simulink library "VolumeMute"  (R2022b)
settings: Solver=VariableStepAuto  StartTime=0.0  StopTime=10.0  RelTol=1e-3
libraries: NonEntGainCalcBtc x4, NonEntVncAppliedBtc x4, FeaturePath x4, MuteBtc x4, AnnVolumeBtc x4, AnnouncementLevelDetection x1, HandyTextFile x1, RTC x1
settings Model: Creator=ak1044356  LastModifiedBy=sa1045272
settings SolverCC: AlgebraicLoopSolver=TrustRegion
settings DebuggingCC: UnconnectedInputMsg=warning  UnconnectedOutputMsg=warning  UnconnectedLineMsg=warning  SFMachineParentedDataDiag=warning  ArithmeticOperatorsInVariantConditions=warning
settings ModelReferenceCC: EnableRefExpFcnMdlSchedulingChecks=on
settings SFSimCC: CustomCodeUndefinedFunction=UseInterfaceOnly

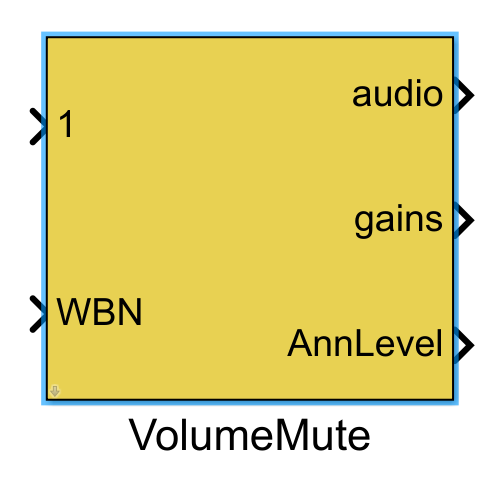
[thumbnail: Simulink's stored preview of the top-level diagram]
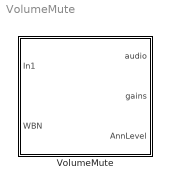
== system VolumeMute ==
  VolumeMute : Subsystem  mask{Config=[]}
      mask prompts: Config "VolumeMuteConfig"
      mask init:
      | blkh=gcbh;
      | Config=BTConfig.Assert(blkh,Config);
      | 
      | Config.Validate();
      | Config.DoMaskInit(blkh);

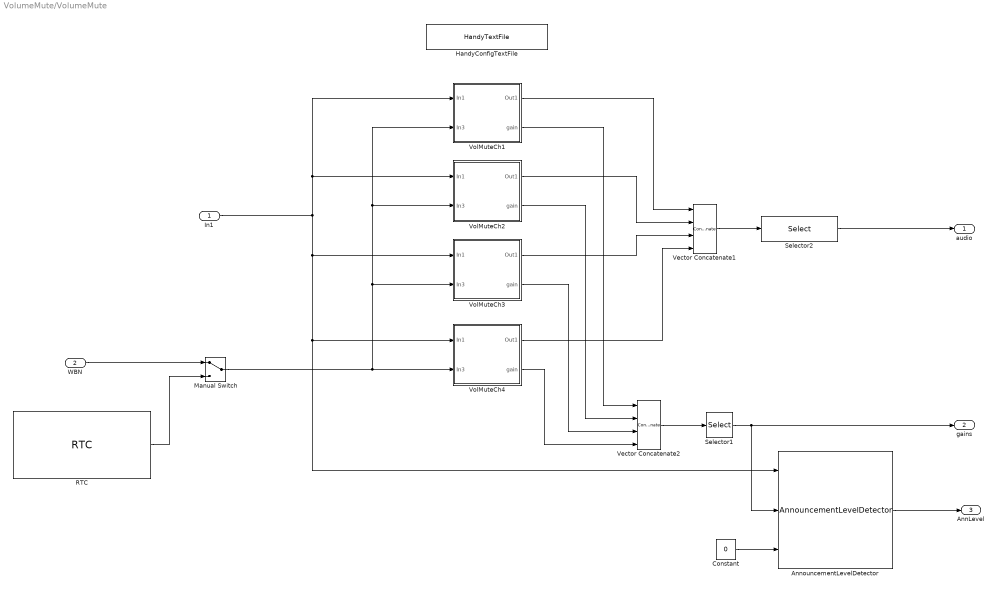
== system VolumeMute/VolumeMute ==
  In1 : Inport
  WBN : Inport  Port=2
  AnnouncementLevelDetector : AnnouncementLevelDetection/AnnouncementLevelDetector  vm=VolumeMuteConfig  DefaultFlag=off  Config=Config.AnnouncementLevelDetector
  Constant : Constant  Value=0
  HandyConfigTextFile : HandyTextFile/HandyTextFile  TemplateSource=Config  FileSuffix=File  OpenDialogOnLoad=off  UseThisBlockName=off  AddGrandParentNamePrefix=off  TheDefaultText=% $(FILENAME) $(PREFIX) $(SUFFIX)  ShowInLibBrowser=on
      settings: SourceProductName=Bose Talaria
  Manual Switch : ManualSwitch
  RTC : RTC/RTC  REQ_Priority=RTC_Mask.NormalPriority  RequestAtInit=off  EnableRequest=off  REQElemName1=NoiseSig  REQElemType1=single  REQElemWidth1=1  REQElemInitial1=NEAR_initial_noise_level  REQElemType2=uint32  REQElemWidth2=1  REQElemInitial2=[]  REQElemType3=uint32  REQElemWidth3=1  REQElemInitial3=[]  REQElemType4=uint32  REQElemWidth4=1  REQElemInitial4=[]  REQElemType5=uint32  REQElemWidth5=1  REQElemInitial5=[]  REQElemType6=uint32  REQElemWidth6=1  REQElemInitial6=[]  REQElemType7=uint32  REQElemWidth7=1  REQElemInitial7=[]  REQElemType8=uint32  REQElemWidth8=1  REQElemInitial8=[]  REQElemType9=uint32  REQElemWidth9=1  REQElemInitial9=[]  REQElemType10=uint32  REQElemWidth10=1  REQElemInitial10=[]  EnableResponse=off  EnableRSP_StatusIn=off  RSPElemType1=uint32  RSPElemWidth1=1  RSPElemType2=uint32  RSPElemWidth2=1  RSPElemType3=uint32  RSPElemWidth3=1  RSPElemType4=uint32  RSPElemWidth4=1  RSPElemType5=uint32  RSPElemWidth5=1  RSPElemType6=uint32  RSPElemWidth6=1  RSPElemType7=uint32  RSPElemWidth7=1  RSPElemType8=uint32  RSPElemWidth8=1  RSPElemType9=uint32  RSPElemWidth9=1  RSPElemType10=uint32  RSPElemWidth10=1  EnableNotification=off  EnableNTF_PrepTrig=off  NTFElemType1=uint32  NTFElemWidth1=1  NTFElemType2=uint32  NTFElemWidth2=1  NTFElemType3=uint32  NTFElemWidth3=1  NTFElemType4=uint32  NTFElemWidth4=1  NTFElemType5=uint32  NTFElemWidth5=1  NTFElemType6=uint32  NTFElemWidth6=1  NTFElemType7=uint32  NTFElemWidth7=1  NTFElemType8=uint32  NTFElemWidth8=1  NTFElemType9=uint32  NTFElemWidth9=1  NTFElemType10=uint32  NTFElemWidth10=1  MaskMessageName=AnnNoiseLevel
      settings: SourceProductName=Bose Talaria
  Selector1 : Selector  NumberOfDimensions=2  InputPortWidth=3  IndexOptions=Select all,Index vector (dialog)  Indices=[1 3],1:Config.AnnChannelCount  OutputSizes=1,1
  Selector2 : Selector  NumberOfDimensions=2  InputPortWidth=3  IndexOptions=Select all,Index vector (dialog)  Indices=[1 3],1:Config.AnnChannelCount  OutputSizes=1,1
  Vector Concatenate1 : Concatenate  NumInputs=4  Mode=Multidimensional array  ConcatenateDimension=2
  Vector Concatenate2 : Concatenate  NumInputs=4  Mode=Multidimensional array  ConcatenateDimension=2
  VolMuteCh1 : Subsystem
  VolMuteCh2 : Subsystem
  VolMuteCh3 : Subsystem
  VolMuteCh4 : Subsystem
  audio : Outport  VectorParamsAs1DForOutWhenUnconnected=off
  gains : Outport  Port=2
  AnnLevel : Outport  Port=3
  wires:
  WBN/1 -> Manual Switch/1
  RTC/1 -> Manual Switch/2
  AnnouncementLevelDetector/1 -> AnnLevel/1
  Constant/1 -> AnnouncementLevelDetector/3
  Selector1/1 -> AnnouncementLevelDetector/2, gains/1
  VolMuteCh4/2(gain) -> Vector Concatenate2/4
  VolMuteCh3/2(gain) -> Vector Concatenate2/3
  VolMuteCh2/2(gain) -> Vector Concatenate2/2
  VolMuteCh1/2(gain) -> Vector Concatenate2/1
  Vector Concatenate2/1 -> Selector1/1
  Manual Switch/1 -> VolMuteCh4/2(In3), VolMuteCh3/2(In3), VolMuteCh2/2(In3), VolMuteCh1/2(In3)
  Selector2/1 -> audio/1
  Vector Concatenate1/1 -> Selector2/1
  In1/1 -> VolMuteCh2/1(In1), VolMuteCh1/1(In1), VolMuteCh3/1(In1), AnnouncementLevelDetector/1, VolMuteCh4/1(In1)
  VolMuteCh1/1(Out1) -> Vector Concatenate1/1
  VolMuteCh3/1(Out1) -> Vector Concatenate1/3
  VolMuteCh4/1(Out1) -> Vector Concatenate1/4
  VolMuteCh2/1(Out1) -> Vector Concatenate1/2

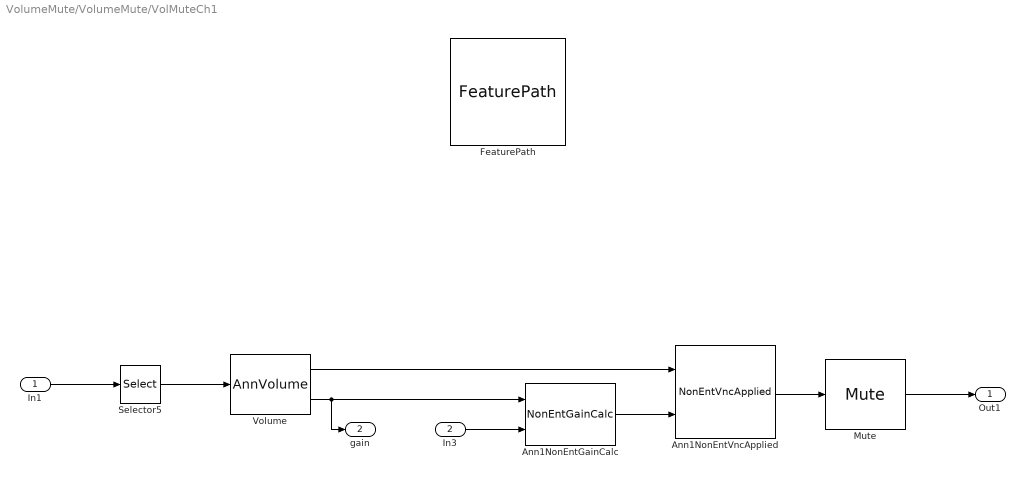
== system VolumeMute/VolumeMute/VolMuteCh1 ==
  In1 : Inport
  In3 : Inport  Port=2
  Ann1NonEntGainCalc : NonEntGainCalcBtc/NonEntGainCalc  Config=Config.Ann1NonEntGainCalc  FeatureName=Ann1NonEntGainCalc
      settings: SourceProductName=Bose Blocklib
  Ann1NonEntVncApplied : NonEntVncAppliedBtc/NonEntVncApplied  Config=Config.Ann1NonEntVncApplied  FeatureName=Ann1NonEntVncApplied
      settings: SourceProductName=Bose Blocklib
  FeaturePath : FeaturePath/FeaturePath  FeatureName=Ann1  IsGroup=off  GroupNumber=-1  IsModule=off  TriggerInit=[270 -291 385 -184]
      settings: SourceProductName=Bose Talaria
  Mute : MuteBtc/Mute  Config=Config.Ann1Mute  FeatureName=Ann1Mute
      settings: SourceProductName=Bose Blocklib
  Selector5 : Selector  NumberOfDimensions=2  InputPortWidth=3  IndexOptions=Select all,Index vector (dialog)  Indices=[1 3],1  OutputSizes=1,1
  Volume : AnnVolumeBtc/AnnVolume  FeatureName=Ann1Volume  Config=Config.Ann1Volume  TriggerInit=[50 25 130 85]
      settings: SourceProductName=Bose Blocklib
  Out1 : Outport  VectorParamsAs1DForOutWhenUnconnected=off
  gain : Outport  Port=2
  wires:
  Mute/1 -> Out1/1
  In1/1 -> Selector5/1
  Selector5/1 -> Volume/1
  In3/1 -> Ann1NonEntGainCalc/2
  Volume/1 -> Ann1NonEntVncApplied/1
  Volume/2 -> Ann1NonEntGainCalc/1, gain/1
  Ann1NonEntVncApplied/1 -> Mute/1
  Ann1NonEntGainCalc/1 -> Ann1NonEntVncApplied/2

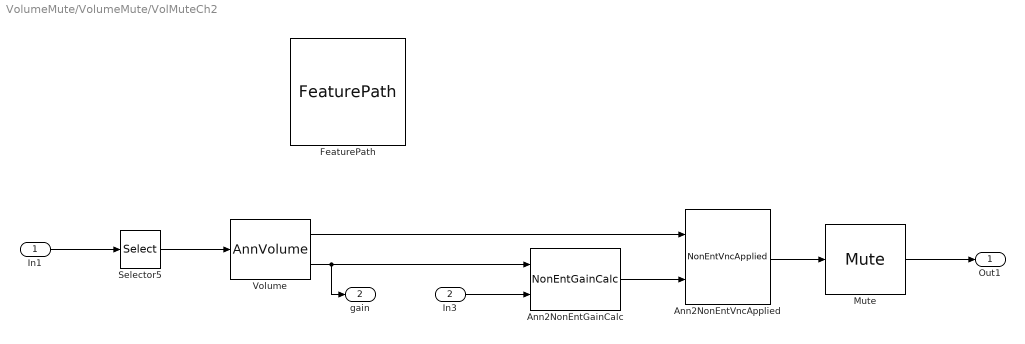
== system VolumeMute/VolumeMute/VolMuteCh2 ==
  In1 : Inport
  In3 : Inport  Port=2
  Ann2NonEntGainCalc : NonEntGainCalcBtc/NonEntGainCalc  Config=Config.Ann2NonEntGainCalc  FeatureName=Ann2NonEntGainCalc
      settings: SourceProductName=Bose Blocklib
  Ann2NonEntVncApplied : NonEntVncAppliedBtc/NonEntVncApplied  Config=Config.Ann2NonEntVncApplied  FeatureName=Ann2NonEntVncApplied
      settings: SourceProductName=Bose Blocklib
  FeaturePath : FeaturePath/FeaturePath  FeatureName=Ann2  IsGroup=off  GroupNumber=-1  IsModule=off  TriggerInit=[60 -206 175 -99]
      settings: SourceProductName=Bose Talaria
  Mute : MuteBtc/Mute  Config=Config.Ann2Mute  FeatureName=Ann2Mute
      settings: SourceProductName=Bose Blocklib
  Selector5 : Selector  NumberOfDimensions=2  InputPortWidth=3  IndexOptions=Select all,Index vector (dialog)  Indices=[1 3],min(2, Config.AnnChannelCount)  OutputSizes=1,1
  Volume : AnnVolumeBtc/AnnVolume  FeatureName=Ann2Volume  Config=Config.Ann2Volume  TriggerInit=[0 -25 80 35]
      settings: SourceProductName=Bose Blocklib
  Out1 : Outport  VectorParamsAs1DForOutWhenUnconnected=off
  gain : Outport  Port=2
  wires:
  Ann2NonEntGainCalc/1 -> Ann2NonEntVncApplied/2
  Ann2NonEntVncApplied/1 -> Mute/1
  Volume/2 -> Ann2NonEntGainCalc/1, gain/1
  Volume/1 -> Ann2NonEntVncApplied/1
  Selector5/1 -> Volume/1
  In1/1 -> Selector5/1
  In3/1 -> Ann2NonEntGainCalc/2
  Mute/1 -> Out1/1

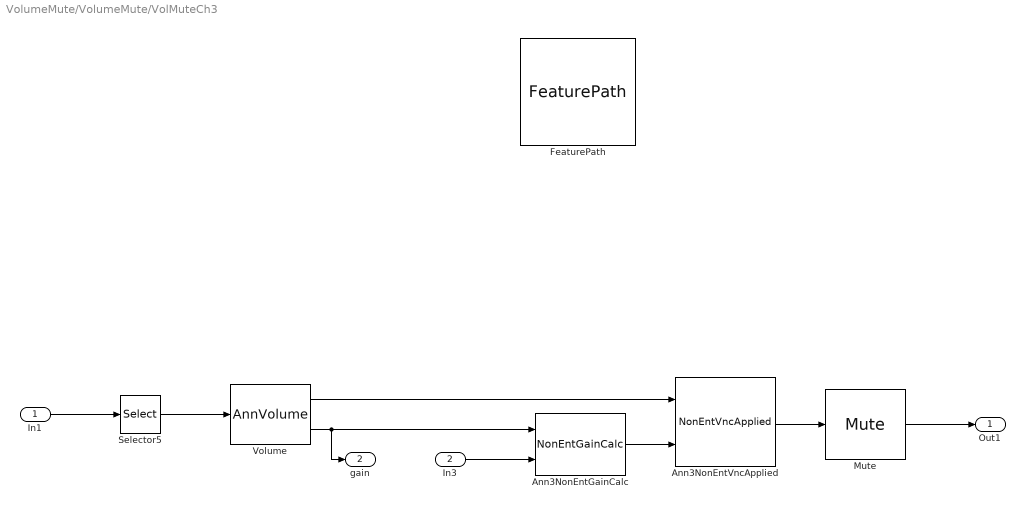
== system VolumeMute/VolumeMute/VolMuteCh3 ==
  In1 : Inport
  In3 : Inport  Port=2
  Ann3NonEntGainCalc : NonEntGainCalcBtc/NonEntGainCalc  Config=Config.Ann3NonEntGainCalc  FeatureName=Ann3NonEntGainCalc
      settings: SourceProductName=Bose Blocklib
  Ann3NonEntVncApplied : NonEntVncAppliedBtc/NonEntVncApplied  Config=Config.Ann3NonEntVncApplied  FeatureName=Ann3NonEntVncApplied
      settings: SourceProductName=Bose Blocklib
  FeaturePath : FeaturePath/FeaturePath  FeatureName=Ann3  IsGroup=off  GroupNumber=-1  IsModule=off  TriggerInit=[265 -336 380 -229]
      settings: SourceProductName=Bose Talaria
  Mute : MuteBtc/Mute  Config=Config.Ann3Mute  FeatureName=Ann3Mute
      settings: SourceProductName=Bose Blocklib
  Selector5 : Selector  NumberOfDimensions=2  InputPortWidth=3  IndexOptions=Select all,Index vector (dialog)  Indices=[1 3],min(3, Config.AnnChannelCount)  OutputSizes=1,1
  Volume : AnnVolumeBtc/AnnVolume  FeatureName=Ann3Volume  Config=Config.Ann3Volume  TriggerInit=[815 415 895 475]
      settings: SourceProductName=Bose Blocklib
  Out1 : Outport  VectorParamsAs1DForOutWhenUnconnected=off
  gain : Outport  Port=2
  wires:
  Ann3NonEntGainCalc/1 -> Ann3NonEntVncApplied/2
  Ann3NonEntVncApplied/1 -> Mute/1
  Volume/2 -> Ann3NonEntGainCalc/1, gain/1
  Volume/1 -> Ann3NonEntVncApplied/1
  Selector5/1 -> Volume/1
  In1/1 -> Selector5/1
  In3/1 -> Ann3NonEntGainCalc/2
  Mute/1 -> Out1/1

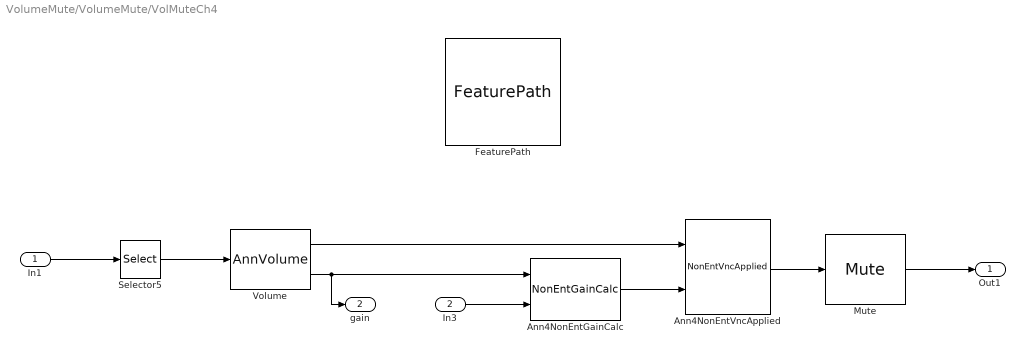
== system VolumeMute/VolumeMute/VolMuteCh4 ==
  In1 : Inport
  In3 : Inport  Port=2
  Ann4NonEntGainCalc : NonEntGainCalcBtc/NonEntGainCalc  Config=Config.Ann4NonEntGainCalc  FeatureName=Ann4NonEntGainCalc
      settings: SourceProductName=Bose Blocklib
  Ann4NonEntVncApplied : NonEntVncAppliedBtc/NonEntVncApplied  Config=Config.Ann4NonEntVncApplied  FeatureName=Ann4NonEntVncApplied
      settings: SourceProductName=Bose Blocklib
  FeaturePath : FeaturePath/FeaturePath  FeatureName=Ann4  IsGroup=off  GroupNumber=-1  IsModule=off  TriggerInit=[235 -186 350 -79]
      settings: SourceProductName=Bose Talaria
  Mute : MuteBtc/Mute  Config=Config.Ann4Mute  FeatureName=Ann4Mute
      settings: SourceProductName=Bose Blocklib
  Selector5 : Selector  NumberOfDimensions=2  InputPortWidth=3  IndexOptions=Select all,Index vector (dialog)  Indices=[1 3],min(4, Config.AnnChannelCount)  OutputSizes=1,1
  Volume : AnnVolumeBtc/AnnVolume  FeatureName=Ann4Volume  Config=Config.Ann4Volume  TriggerInit=[20 5 100 65]
      settings: SourceProductName=Bose Blocklib
  Out1 : Outport  VectorParamsAs1DForOutWhenUnconnected=off
  gain : Outport  Port=2
  wires:
  Ann4NonEntGainCalc/1 -> Ann4NonEntVncApplied/2
  Ann4NonEntVncApplied/1 -> Mute/1
  Volume/2 -> Ann4NonEntGainCalc/1, gain/1
  Volume/1 -> Ann4NonEntVncApplied/1
  Selector5/1 -> Volume/1
  In1/1 -> Selector5/1
  In3/1 -> Ann4NonEntGainCalc/2
  Mute/1 -> Out1/1
